simulink model "diffur"  (R2019a)
settings: Solver=VariableStepAuto  StartTime=0.0  StopTime=10.0  RelTol=1e-3
libraries: simulink x1
settings Model: Creator=step_oda  LastModifiedBy=bomjz
settings DataIOCC: ReturnWorkspaceOutputs=off
settings DebuggingCC: ArithmeticOperatorsInVariantConditions=warning
settings SFSimCC: SimUseLocalCustomCode=off
settings RTWCC: RTWUseLocalCustomCode=off
settings CodeAppCC: StateflowObjectComments=on

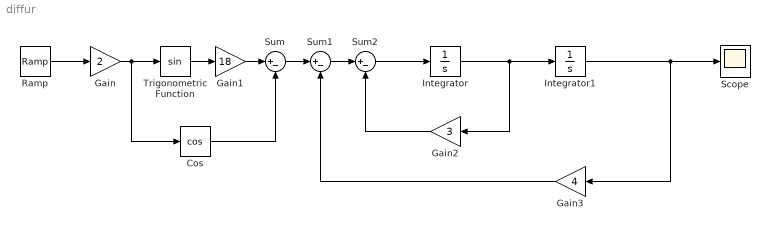
== system diffur ==
  Cos : Trigonometry  Operator=cos
  Gain : Gain  Gain=2
  Gain1 : Gain  Gain=18
  Gain2 : Gain  Gain=3
  Gain3 : Gain  Gain=4
  Integrator : Integrator  InitialCondition=1
  Integrator1 : Integrator
  Ramp : simulink/Sources/Ramp  slope=1  start=0  InitialOutput=0
  Scope : Scope
  Sum : Sum  Inputs=|+-
  Sum1 : Sum  Inputs=|+-
  Sum2 : Sum  Inputs=|+-
  Trigonometric Function : Trigonometry
  wires:
  Ramp/1 -> Gain/1
  Gain/1 -> Cos/1, Trigonometric Function/1
  Sum1/1 -> Sum2/1
  Sum/1 -> Sum1/1
  Trigonometric Function/1 -> Gain1/1
  Sum2/1 -> Integrator/1
  Integrator/1 -> Gain2/1, Integrator1/1
  Integrator1/1 -> Gain3/1, Scope/1
  Gain2/1 -> Sum2/2
  Gain3/1 -> Sum1/2
  Cos/1 -> Sum/2
  Gain1/1 -> Sum/1
